simulink model "IEEE13NodeTestFeeder"  (R2024a)
settings: Solver=ode45  StartTime=0.0  StopTime=0.2  MaxStep=0.04  RelTol=1e-3
PreLoadFcn:
  | IEEE13NodeTestFeederInit;
  | Ts=50e-6
undefined symbols (not defined in the file or in its folder): C_601, C_602, C_603, C_604, C_605, C_606, C_607, ft2km, L_601, L_602, L_603, L_604, L_605, L_606, L_607, R_601, R_602, R_603, R_604, R_605, R_606, R_607
libraries: spsLoadFlowBusLib x12, spsPiSectionLineLib x9, spsThreePhaseSeriesRLCLoadLib x7, spsThreePhaseDynamicLoadLib x6, spsGroundLib x6, spsMultimeterLib x6, spsPowerPhasorLib x6, spsSeriesRLCLoadLib x5, spsThreePhaseVIMeasurementLib x4, spsThreePhaseSourceLib x1, spsThreePhaseBreakerLib x1, spsThreePhaseTransformerTwoWindingsLib x1
settings Model: Creator=The MathWorks, Inc.  LastModifiedBy=ethan
settings SolverCC: AlgebraicLoopSolver=TrustRegion
settings DataIOCC: ExternalInput=getinputstruct(op_IEEE_13_node_5)  InitialState=getstatestruct(op_IEEE_13_node_5)  LimitDataPoints=on  SaveFormat=Array  ReturnWorkspaceOutputs=off
settings OptimizationCC: LifeSpan=inf
settings DebuggingCC: AlgebraicLoopMsg=none  FcnCallInpInsideContextMsg=warning  StateNameClashWarn=warning  SFUnexpectedBacktrackingDiag=warning  SFNoUnconditionalDefaultTransitionDiag=warning  SFExecutionAtInitializationDiag=none
settings ModelReferenceCC: EnableRefExpFcnMdlSchedulingChecks=on  PropagateSignalLabelsOutOfModel=off
settings SFSimCC: CustomCodeUndefinedFunction=UseInterfaceOnly
settings RTWCC: GPUComputeCapability=3.5
settings CodeAppCC: StateflowObjectComments=on
settings SimscapeCC: SimscapeNormalizeSystem=off

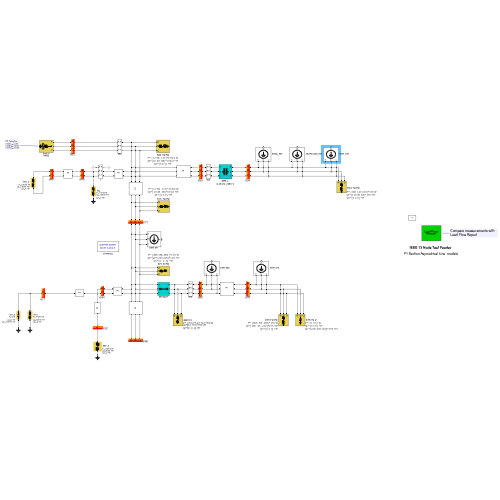
[thumbnail: Simulink's stored preview of the top-level diagram]
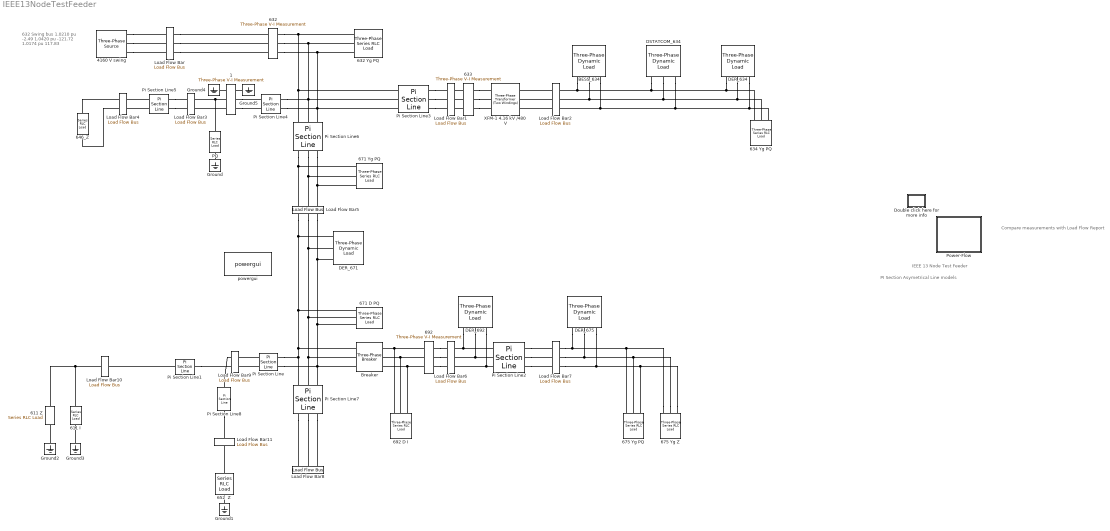
== system IEEE13NodeTestFeeder ==
  note: Compare measurements with
      | Load Flow Report
  note: 632 Swing bus
      | 1.0210 pu -2.49
      | 1.0420 pu -121.72
      | 1.0174 pu 117.83
  note: PI Section Asymetrical Line models
  note: IEEE 13 Node Test Feeder
  " 634 Yg PQ " : spsThreePhaseSeriesRLCLoadLib/Three-Phase Series RLC Load  LConnTagsString=A|B|C  Configuration=Y (grounded)  NominalVoltage=120e3  Vabc=[ 1.04003 1.06954 1.04523]*277.128  Vabcp=[1e3 1e3 1e3]  NominalFrequency=60  UnbalancedPower=on  ActivePower=1e+006  InductivePower=0  CapacitivePower=0  Pabc=[160 120 120]*1e3  QLabc=[110 90 90]*1e3  QCabc=[0 0 0]  Pabcp=[10e3 9e3 11e3]  QLabcp=[100 90 110]  QCabcp=[100 90 110]  Measurements=None  LoadType=constant PQ
      settings: AttributesFormatString=|
      | P= %<Pabc> W
      | Ql=%<QLabc> var
      | Qc=%<QCabc> var
  1 : spsThreePhaseVIMeasurementLib/Three-Phase V-I Measurement  VoltageMeasurement=phase-to-ground  SetLabelV=on  LabelV=Vabc_645  Vpu=off  VpuLL=off  CurrentMeasurement=yes  SetLabelI=on  LabelI=Iabc_645  Ipu=off  Pbase=100e6  Vbase=4160  OutputType=Complex  PhasorSimulation=on  PSBequivalent=0
  4160 V swing : spsThreePhaseSourceLib/Three-Phase Source  InternalConnection=Yg  VoltagePhases=on  Voltage=120e3  PhaseAngle=0  Voltage_phases=[ 1.021 1.042 1.0174]*2401.78  PhaseAngles_phases=[ -2.49008 -121.72 117.83]  Frequency=60  NonIdealSource=on  SpecifyImpedance=off  Resistance=1e-5  Inductance=0  ShortCircuitLevel=100e6  BaseVoltage=120e3  XRratio=10  BusType=swing  Pref=0  Qref=0  Prefabc=[0 0 0]  Qrefabc=[0 0 0]  Qmin="[-inf  -inf -inf]"  Qmax="[inf  inf inf]"
  611 I : spsSeriesRLCLoadLib/Series RLC Load  LConnTagsString=a  RConnTagsString=__new0  NominalVoltage=0.986755*2401.78  NominalFrequency=60  ActivePower=170e3  InductivePower=80e3  CapacitivePower=0  Setx0=off  InitialVoltage=0  SetiL0=off  InitialCurrent=0  Measurements=Branch voltage and current  LoadType=constant I
      settings: AttributesFormatString=|
      | P=%<ActivePower> W
      | Ql=%<InductivePower> var
      | Qc=%<CapacitivePower> var
  611 Z : spsSeriesRLCLoadLib/Series RLC Load  LConnTagsString=a  RConnTagsString=__new0  NominalVoltage=4160/sqrt(3)  NominalFrequency=60  ActivePower=0  InductivePower=0  CapacitivePower=100e3  Setx0=off  InitialVoltage=0  SetiL0=off  InitialCurrent=0  Measurements=None  LoadType=constant Z
      settings: AttributesFormatString=|
      | P=%<ActivePower> W
      | Ql=%<InductivePower> var
      | Qc=%<CapacitivePower> var
  632 : spsThreePhaseVIMeasurementLib/Three-Phase V-I Measurement  VoltageMeasurement=phase-to-ground  SetLabelV=on  LabelV=Vabc_632  Vpu=off  VpuLL=off  CurrentMeasurement=yes  SetLabelI=on  LabelI=Iabc_632  Ipu=off  Pbase=100e6  Vbase=4160  OutputType=Complex  PhasorSimulation=on  PSBequivalent=0
  632 Yg PQ : spsThreePhaseSeriesRLCLoadLib/Three-Phase Series RLC Load  LConnTagsString=A|B|C  Configuration=Y (grounded)  NominalVoltage=120e3  Vabc=[ 1.021 1.042 1.0174]*2401.78  Vabcp=[1e3 1e3 1e3]  NominalFrequency=60  UnbalancedPower=on  ActivePower=1e+006  InductivePower=0  CapacitivePower=0  Pabc="[17 66  117]*1e3/2"  QLabc="[10 38  68]*1e3/2"  QCabc=[0 0 0]  Pabcp=[10e3 9e3 11e3]  QLabcp=[100 90 110]  QCabcp=[100 90 110]  Measurements=None  LoadType=constant PQ
      settings: AttributesFormatString=|
      | P= %<Pabc> W
      | Ql=%<QLabc> var
      | Qc=%<QCabc> var
  633 : spsThreePhaseVIMeasurementLib/Three-Phase V-I Measurement  VoltageMeasurement=phase-to-ground  SetLabelV=on  LabelV=Vabc_633  Vpu=off  VpuLL=off  CurrentMeasurement=yes  SetLabelI=on  LabelI=Iabc_633  Ipu=off  Pbase=100e6  Vbase=4160  OutputType=Complex  PhasorSimulation=on  PSBequivalent=0
  646_Z : spsSeriesRLCLoadLib/Series RLC Load  LConnTagsString=a  RConnTagsString=__new0  NominalVoltage=4160  NominalFrequency=60  ActivePower=230e3  InductivePower=132e3  CapacitivePower=0  Setx0=off  InitialVoltage=0  SetiL0=off  InitialCurrent=0  Measurements=None  LoadType=constant Z
      settings: AttributesFormatString=|
      | P=%<ActivePower> W
      | Ql=%<InductivePower> var
      | Qc=%<CapacitivePower> var
  "652  Z " : spsSeriesRLCLoadLib/Series RLC Load  LConnTagsString=a  RConnTagsString=__new0  NominalVoltage=4160/sqrt(3)  NominalFrequency=60  ActivePower=128e3  InductivePower=86e3  CapacitivePower=0  Setx0=off  InitialVoltage=0  SetiL0=off  InitialCurrent=0  Measurements=None  LoadType=constant Z
      settings: AttributesFormatString=|
      | P=%<ActivePower> W
      | Ql=%<InductivePower> var
      | Qc=%<CapacitivePower> var
  671 D PQ : spsThreePhaseSeriesRLCLoadLib/Three-Phase Series RLC Load  LConnTagsString=A|B|C  Configuration=Delta  NominalVoltage=120e3  Vabc="[1  1  1]*120e3/sqrt(3)"  Vabcp=[ 1.7426 1.77325 1.71534]*2401.78  NominalFrequency=60  UnbalancedPower=on  ActivePower=1e+006  InductivePower=0  CapacitivePower=0  Pabc="[17 66  117]*1e3/2"  QLabc="[10 38  68]*1e3/2"  QCabc=[0 0 0]  Pabcp=[385 385 385 ]*1e3  QLabcp=[220 220 220]*1e3  QCabcp="[0  0  0]"  Measurements=Branch voltages and currents  LoadType=constant PQ
      settings: AttributesFormatString=|
      | P= %<Pabcp> W
      | Ql=%<QLabcp> var
      | Qc=%<QCabcp> var
  671 Yg PQ : spsThreePhaseSeriesRLCLoadLib/Three-Phase Series RLC Load  LConnTagsString=A|B|C  Configuration=Y (grounded)  NominalVoltage=120e3  Vabc=[ 0.990007 1.05293 0.977696]*2401.78  Vabcp=[1e3 1e3 1e3]  NominalFrequency=60  UnbalancedPower=on  ActivePower=1e+006  InductivePower=0  CapacitivePower=0  Pabc="[17 66  117]*1e3/2"  QLabc="[10 38  68]*1e3/2"  QCabc=[0 0 0]  Pabcp=[10e3 9e3 11e3]  QLabcp=[100 90 110]  QCabcp=[100 90 110]  Measurements=None  LoadType=constant PQ
      settings: AttributesFormatString=|
      | P= %<Pabc> W
      | Ql=%<QLabc> var
      | Qc=%<QCabc> var
  675 Yg PQ : spsThreePhaseSeriesRLCLoadLib/Three-Phase Series RLC Load  LConnTagsString=A|B|C  Configuration=Y (grounded)  NominalVoltage=120e3  Vabc=[ 0.983621 1.05532 0.975578]*2401.78  Vabcp=[1e3 1e3 1e3]  NominalFrequency=60  UnbalancedPower=on  ActivePower=1e+006  InductivePower=0  CapacitivePower=0  Pabc="[485  68  290]*1e3"  QLabc="[190  60  212]*1e3"  QCabc=[0 0 0]  Pabcp=[10e3 9e3 11e3]  QLabcp=[100 90 110]  QCabcp=[100 90 110]  Measurements=Branch voltages and currents  LoadType=constant PQ
      settings: AttributesFormatString=|
      | P= %<Pabc> W
      | Ql=%<QLabc> var
      | Qc=%<QCabc> var
  675 Yg Z : spsThreePhaseSeriesRLCLoadLib/Three-Phase Series RLC Load  LConnTagsString=A|B|C  Configuration=Y (grounded)  NominalVoltage=120e3  Vabc="[1  1  1]*4160/sqrt(3)"  Vabcp=[1e3 1e3 1e3]  NominalFrequency=60  UnbalancedPower=on  ActivePower=1e+006  InductivePower=0  CapacitivePower=0  Pabc=[0 0 0]  QLabc=[0 0 0]  QCabc=[200 200 200]*1e3  Pabcp=[10e3 9e3 11e3]  QLabcp=[100 90 110]  QCabcp=[100 90 110]  Measurements=None  LoadType=constant Z
      settings: AttributesFormatString=|
      | P= %<Pabc> W
      | Ql=%<QLabc> var
      | Qc=%<QCabc> var
  692 : spsThreePhaseVIMeasurementLib/Three-Phase V-I Measurement  VoltageMeasurement=phase-to-ground  SetLabelV=on  LabelV=Vabc_692  Vpu=off  VpuLL=off  CurrentMeasurement=yes  SetLabelI=on  LabelI=Iabc_692  Ipu=off  Pbase=100e6  Vbase=4160  OutputType=Complex  PhasorSimulation=on  PSBequivalent=0
  692 D I : spsThreePhaseSeriesRLCLoadLib/Three-Phase Series RLC Load  LConnTagsString=A|B|C  Configuration=Delta  NominalVoltage=120e3  Vabc="[1  1  1]*120e3/sqrt(3)"  Vabcp=[ 1.73731 1.75253 1.72367]*2401.78  NominalFrequency=60  UnbalancedPower=on  ActivePower=1e+006  InductivePower=0  CapacitivePower=0  Pabc="[17 66  117]*1e3/2"  QLabc="[10 38  68]*1e3/2"  QCabc=[0 0 0]  Pabcp=[1e-6 1e-6 170 ]*1e3  QLabcp=[0 0 151]*1e3  QCabcp="[0  0  0]"  Measurements=Branch voltages and currents  LoadType=constant I
      settings: AttributesFormatString=|
      | P= %<Pabcp> W
      | Ql=%<QLabcp> var
      | Qc=%<QCabcp> var
  BESS_634 : spsThreePhaseDynamicLoadLib/Three-Phase Dynamic Load  NominalVoltage=[4160 60]  ActiveReactivePowers=[0 0]  PositiveSequence=[0.121336 5.51821]  ExternalControl=off  NpNq=[0 0]  TimeConstants="[0  0  0  0]"  MinimumVoltage=0.7  Tfilter=1e-4  LoadFlowParameters=[4,0,0,0,0]
      settings: LibrarySourceBlock=|
      | sps_lib/Passives/Three-Phase
      | Dynamic Load
  Breaker : spsThreePhaseBreakerLib/Three-Phase Breaker  InitialState=closed  SwitchA=off  SwitchB=off  SwitchC=off  SwitchTimes=[0.5 ]  External=off  BreakerResistance=0.0001  SnubberResistance=inf  SnubberCapacitance=0  Measurements=None
  DER_634 : spsThreePhaseDynamicLoadLib/Three-Phase Dynamic Load  NominalVoltage=[4160 60]  ActiveReactivePowers=[0 0]  PositiveSequence=[0.121336 5.51821]  ExternalControl=off  NpNq=[0 0]  TimeConstants="[0  0  0  0]"  MinimumVoltage=0.7  Tfilter=1e-4  LoadFlowParameters=[4,0,0,0,0]
      settings: LibrarySourceBlock=|
      | sps_lib/Passives/Three-Phase
      | Dynamic Load
  DER_671 : spsThreePhaseDynamicLoadLib/Three-Phase Dynamic Load  NominalVoltage=[4160 60]  ActiveReactivePowers=[0 0]  PositiveSequence=[1.00665 -3.83837]  ExternalControl=off  NpNq=[0 0]  TimeConstants="[0  0  0  0]"  MinimumVoltage=0.7  Tfilter=1e-4  LoadFlowParameters=[4,0,0,0,0]
      settings: LibrarySourceBlock=|
      | sps_lib/Passives/Three-Phase
      | Dynamic Load
  DER_675 : spsThreePhaseDynamicLoadLib/Three-Phase Dynamic Load  NominalVoltage=[4160 60]  ActiveReactivePowers=[0 0]  PositiveSequence=[1.0046 -3.96901]  ExternalControl=off  NpNq=[0 0]  TimeConstants="[0  0  0  0]"  MinimumVoltage=0.7  Tfilter=1e-4  LoadFlowParameters=[4,0,0,0,0]
      settings: LibrarySourceBlock=|
      | sps_lib/Passives/Three-Phase
      | Dynamic Load
  DER_692 : spsThreePhaseDynamicLoadLib/Three-Phase Dynamic Load  NominalVoltage=[4160 60]  ActiveReactivePowers=[0 0]  PositiveSequence=[1.00665 -3.83836]  ExternalControl=off  NpNq=[0 0]  TimeConstants="[0  0  0  0]"  MinimumVoltage=0.7  Tfilter=1e-4  LoadFlowParameters=[4,0,0,0,0]
      settings: LibrarySourceBlock=|
      | sps_lib/Passives/Three-Phase
      | Dynamic Load
  DSTATCOM_634 : spsThreePhaseDynamicLoadLib/Three-Phase Dynamic Load  NominalVoltage=[4160 60]  ActiveReactivePowers=[0 0]  PositiveSequence=[0.121336 5.51821]  ExternalControl=off  NpNq=[0 0]  TimeConstants="[0  0  0  0]"  MinimumVoltage=0.7  Tfilter=1e-4  LoadFlowParameters=[4,0,0,0,0]
      settings: LibrarySourceBlock=|
      | sps_lib/Passives/Three-Phase
      | Dynamic Load
  Double click here for more info : Subsystem
      settings: OpenFcn="showExample(\"simscapeelectricalsps/IEEE13NodeTestFeederExample\")"
      mask Display: disp('?')
  Ground{,1..5} (6 alike) : spsGroundLib/Ground  LConnTagsString=a
  Load Flow Bar : spsLoadFlowBusLib/Load Flow Bus  LConnTagsString=a|b|c  RConnTagsString=a|b|c  Phases=ABC  Connectors=on both sides  ID=632  Vbase=4160/sqrt(3)  Vref="[ 1.0210  1.0420  1.0174]"  Vangle="[ -2.49  -121.72  117.83]"  VLF=1.021  VLFb=1.042  VLFc=1.017  angleLF=-2.49  angleLFb=-121.7  angleLFc=117.8
      settings: AttributesFormatString=%<ID>
  Load Flow Bar1 : spsLoadFlowBusLib/Load Flow Bus  LConnTagsString=a|b|c  RConnTagsString=a|b|c  Phases=ABC  Connectors=on both sides  ID=633  Vbase=4160/sqrt(3)  Vref=[1.0 1.0 1.0]  Vangle=[0 -120 120]  VLF=1.023  VLFb=1.046  VLFc=1.023  angleLF=-1.782  angleLFb=-120.9  angleLFc=118.7
      settings: AttributesFormatString=%<ID>
  Load Flow Bar10 : spsLoadFlowBusLib/Load Flow Bus  LConnTagsString=a  RConnTagsString=a  Phases=C  Connectors=on both sides  ID=611  Vbase=4160/sqrt(3)  Vref=1.0  Vangle=0  VLF=NaN  VLFb=NaN  VLFc=0.9737  angleLF=NaN  angleLFb=NaN  angleLFc=115.8
      settings: AttributesFormatString=%<ID>
  Load Flow Bar11 : spsLoadFlowBusLib/Load Flow Bus  LConnTagsString=a  RConnTagsString=a  Phases=A  Connectors=on both sides  ID=652  Vbase=4160/sqrt(3)  Vref=1.0  Vangle=0  VLF=0.9825  VLFb=NaN  VLFc=NaN  angleLF=-5.246  angleLFb=NaN  angleLFc=NaN
      settings: AttributesFormatString=%<ID>
  Load Flow Bar2 : spsLoadFlowBusLib/Load Flow Bus  LConnTagsString=a|b|c  RConnTagsString=a|b|c  Phases=ABC  Connectors=on both sides  ID=634  Vbase=480/sqrt(3)  Vref=[1.0 1.0 1.0]  Vangle=[0 -120 120]  VLF=1.04  VLFb=1.07  VLFc=1.045  angleLF=5.014  angleLFb=-114.1  angleLFc=125.6
      settings: AttributesFormatString=%<ID>
  Load Flow Bar3 : spsLoadFlowBusLib/Load Flow Bus  LConnTagsString=a|b  RConnTagsString=a|b  Phases=BC  Connectors=on both sides  ID=645  Vbase=4160/sqrt(3)  Vref=[1.0 1.0 ]  Vangle=[0 0]  VLF=NaN  VLFb=1.033  VLFc=1.015  angleLF=NaN  angleLFb=-121.9  angleLFc=117.9
      settings: AttributesFormatString=%<ID>
  Load Flow Bar4 : spsLoadFlowBusLib/Load Flow Bus  LConnTagsString=a|b  RConnTagsString=a|b  Phases=BC  Connectors=on both sides  ID=646  Vbase=4160/sqrt(3)  Vref=[1.0 1.0 ]  Vangle=[0 0]  VLF=NaN  VLFb=1.031  VLFc=1.013  angleLF=NaN  angleLFb=-122  angleLFc=117.9
      settings: AttributesFormatString=%<ID>
  Load Flow Bar5 : spsLoadFlowBusLib/Load Flow Bus  LConnTagsString=a|b|c  RConnTagsString=a|b|c  Phases=ABC  Connectors=on both sides  ID=671  Vbase=4160/sqrt(3)  Vref=[1.0 1.0 1.0]  Vangle=[0 -120 120]  VLF=0.99  VLFb=1.053  VLFc=0.9777  angleLF=-5.298  angleLFb=-122.3  angleLFc=116
      settings: AttributesFormatString=%<ID>
  Load Flow Bar6 : spsLoadFlowBusLib/Load Flow Bus  LConnTagsString=a|b|c  RConnTagsString=a|b|c  Phases=ABC  Connectors=on both sides  ID=692  Vbase=4160/sqrt(3)  Vref=[1.0 1.0 1.0]  Vangle=[0 -120 120]  VLF=0.99  VLFb=1.053  VLFc=0.9777  angleLF=-5.298  angleLFb=-122.3  angleLFc=116
      settings: AttributesFormatString=%<ID>
  Load Flow Bar7 : spsLoadFlowBusLib/Load Flow Bus  LConnTagsString=a|b|c  RConnTagsString=a|b|c  Phases=ABC  Connectors=on both sides  ID=675  Vbase=4160/sqrt(3)  Vref=[1.0 1.0 1.0]  Vangle=[0 -120 120]  VLF=0.9836  VLFb=1.055  VLFc=0.9756  angleLF=-5.544  angleLFb=-122.5  angleLFc=116
      settings: AttributesFormatString=%<ID>
  Load Flow Bar8 : spsLoadFlowBusLib/Load Flow Bus  LConnTagsString=a|b|c  Phases=ABC  Connectors=on one side  ID=680  Vbase=4160/sqrt(3)  Vref=[1.0 1.0 1.0]  Vangle=[0 -120 120]  VLF=0.99  VLFb=1.053  VLFc=0.9777  angleLF=-5.298  angleLFb=-122.3  angleLFc=116
      settings: AttributesFormatString=%<ID>
  Load Flow Bar9 : spsLoadFlowBusLib/Load Flow Bus  LConnTagsString=a|b  RConnTagsString=a|b  Phases=AC  Connectors=on both sides  ID=684  Vbase=4160/sqrt(3)  Vref=[1.0 1.0 ]  Vangle=[0 -120 ]  VLF=0.9881  VLFb=NaN  VLFc=0.9757  angleLF=-5.321  angleLFb=NaN  angleLFc=115.9
      settings: AttributesFormatString=%<ID>
  PQ : spsSeriesRLCLoadLib/Series RLC Load  LConnTagsString=a  RConnTagsString=__new0  NominalVoltage=1.03283*2401.78  NominalFrequency=60  ActivePower=170e3  InductivePower=125e3  CapacitivePower=0  Setx0=off  InitialVoltage=0  SetiL0=off  InitialCurrent=0  Measurements=None  LoadType=constant PQ
      settings: AttributesFormatString=|
      | P=%<ActivePower> W
      | Ql=%<InductivePower> var
      | Qc=%<CapacitivePower> var
  Pi Section Line : spsPiSectionLineLib/Pi Section Line  LConnTagsString=1|i2  RConnTagsString=1|o2  Phases=2  PiSections=1  Length=300*ft2km  Frequency=60  Resistance=R_604([1 3],[1 3])  Inductance=L_604([1 3],[1 3])  Capacitance=C_604([1 3],[1 3])  SpecifyConductance=off  Conductance=0  Measurements=None  Measurements2=None
      settings: LibrarySourceBlock=sps_lib/Power Grid Elements/Pi Section Line
  Pi Section Line1 : spsPiSectionLineLib/Pi Section Line  LConnTagsString=1  RConnTagsString=1  Phases=1  PiSections=1  Length=300*ft2km  Frequency=60  Resistance=R_605(3,3)  Inductance=L_605(3,3)  Capacitance=C_605(3,3)  SpecifyConductance=off  Conductance=0  Measurements=None  Measurements2=None
      settings: LibrarySourceBlock=sps_lib/Power Grid Elements/Pi Section Line
  Pi Section Line2 : spsPiSectionLineLib/Pi Section Line  LConnTagsString=1|i2|i3  RConnTagsString=1|o2|o3  Phases=3  PiSections=1  Length=500*ft2km  Frequency=60  Resistance=R_606  Inductance=L_606  Capacitance=C_606  SpecifyConductance=off  Conductance=0  Measurements=None  Measurements2=None
      settings: LibrarySourceBlock=sps_lib/Power Grid Elements/Pi Section Line
  Pi Section Line3 : spsPiSectionLineLib/Pi Section Line  LConnTagsString=1|i2|i3  RConnTagsString=1|o2|o3  Phases=3  PiSections=1  Length=500*ft2km  Frequency=60  Resistance=R_602  Inductance=L_602  Capacitance=C_602  SpecifyConductance=off  Conductance=0  Measurements=None  Measurements2=None
      settings: LibrarySourceBlock=sps_lib/Power Grid Elements/Pi Section Line
  Pi Section Line4 : spsPiSectionLineLib/Pi Section Line  LConnTagsString=1|i2  RConnTagsString=1|o2  Phases=2  PiSections=1  Length=500*ft2km  Frequency=60  Resistance=R_603(2:3,2:3)  Inductance=L_603(2:3,2:3)  Capacitance=C_603(2:3,2:3)  SpecifyConductance=off  Conductance=0  Measurements=None  Measurements2=None
      settings: LibrarySourceBlock=sps_lib/Power Grid Elements/Pi Section Line
  Pi Section Line5 : spsPiSectionLineLib/Pi Section Line  LConnTagsString=1|i2  RConnTagsString=1|o2  Phases=2  PiSections=1  Length=300*ft2km  Frequency=60  Resistance=R_603(2:3,2:3)  Inductance=L_603(2:3,2:3)  Capacitance=C_603(2:3,2:3)  SpecifyConductance=off  Conductance=0  Measurements=None  Measurements2=None
      settings: LibrarySourceBlock=sps_lib/Power Grid Elements/Pi Section Line
  Pi Section Line6 : spsPiSectionLineLib/Pi Section Line  LConnTagsString=1|i2|i3  RConnTagsString=1|o2|o3  Phases=3  PiSections=1  Length=2000*ft2km  Frequency=60  Resistance=R_601  Inductance=L_601  Capacitance=C_601  SpecifyConductance=off  Conductance=0  Measurements=None  Measurements2=None
      settings: LibrarySourceBlock=sps_lib/Power Grid Elements/Pi Section Line
  Pi Section Line7 : spsPiSectionLineLib/Pi Section Line  LConnTagsString=1|i2|i3  RConnTagsString=1|o2|o3  Phases=3  PiSections=1  Length=1000*ft2km  Frequency=60  Resistance=R_601  Inductance=L_601  Capacitance=C_601  SpecifyConductance=off  Conductance=0  Measurements=None  Measurements2=None
      settings: LibrarySourceBlock=sps_lib/Power Grid Elements/Pi Section Line
  Pi Section Line8 : spsPiSectionLineLib/Pi Section Line  LConnTagsString=1  RConnTagsString=1  Phases=1  PiSections=1  Length=800*ft2km  Frequency=60  Resistance=R_607(1,1)  Inductance=L_607(1,1)  Capacitance=C_607(1,1)  SpecifyConductance=off  Conductance=0  Measurements=None  Measurements2=None
      settings: LibrarySourceBlock=sps_lib/Power Grid Elements/Pi Section Line
  Power-Flow : Subsystem
      mask Display: disp('Load Flow\nResults')
  XFM-1 4.16 kV /480 V : spsThreePhaseTransformerTwoWindingsLib/Three-Phase Transformer (Two Windings)  Winding1Connection=Yg  Winding2Connection=Yg  CoreType=Three single-phase transformers  SetSaturation=off  Hysteresis=off  DataFile='hysteresis'  SetInitialFlux=off  Measurements=None  UNITS=pu  NominalPower=[ 500e3 , 60 ]  Winding1=[4160 0.011 0.02]  Winding2=[480 0 0]  Rm=500  Lm=500  L0=0.5  Saturation=[0 0;0.0024 1.2;1 1.52]  InitialFluxes=[0.8 -0.8 0.7]  BreakLoop=off  DiscreteSolver=Trapezoidal iterative  DataType=off  TransfoNumber=1
  powergui : spspowerguiLib/powergui  Priority=1  SimulationMode=Discrete phasor  SampleTime=4e-3  frequency=60  Iterations=50  frequencyindice=60  Pbase=100e3  ErrMax=0.0001  UnitsV=kV  UnitsW=kW  buscounter=0  FunctionMessages=off  echomessages=off  EnableUseOfTLC=off  CurrentSourceSwitches=off  DisableSnubberDevices=off  DisableRonSwitches=off  DisableVfSwitches=off  DisplayEquations=off  AutomaticDiscreteSolvers=off  SolverType=Tustin/Backward Euler (TBE)  Interpol=off  ExternalGateDelay=off  methode=off  Ts=0  x0status=blocks  SPID=off  SwTol=0  HookPort=off  NonlinearTolerance=1e-4  nMaxIteration=100  ContinueOnMaxIteration=off  RestoreLinks=warning  ResistiveCurrentMeasurement=off  Frange=[0:2:500]  Ylog=off  Xlog=on  ShowGrid=off  save=off  variable=ZData  structure=0  ZoomFFT=on  StartTime=0.0  cycles=1  DisplayStyle=1  fundamental=60  FreqAxis=off  MaxFrequency=1000  frequencyindicesteady=1  RmsSteady=1  display=off
  connections:
  632/RConn2 -- 632 Yg PQ/LConn2 -- Pi Section Line4/RConn1 -- Pi Section Line6/LConn2 -- Pi Section Line3/LConn2
  675 Yg Z/LConn1 -- DER_675/LConn1 -- Load Flow Bar7/LConn1 -- 675 Yg PQ/LConn1
  671 D PQ/LConn2 -- DER_671/LConn2 -- Load Flow Bar5/RConn2 -- Breaker/LConn2 -- Pi Section Line7/LConn2
  Breaker/RConn3 -- 692 D I/LConn3 -- 692/LConn3
  Pi Section Line/RConn1 -- Pi Section Line7/LConn1 -- DER_671/LConn1 -- Load Flow Bar5/RConn1 -- 671 D PQ/LConn1 -- Breaker/LConn1
  Load Flow Bar3/RConn1 -- 1/LConn2 -- PQ/LConn1
  675 Yg Z/LConn3 -- DER_675/LConn3 -- Load Flow Bar7/LConn3 -- 675 Yg PQ/LConn3
  671 Yg PQ/LConn2 -- Load Flow Bar5/LConn2 -- Pi Section Line6/RConn2
  611 I/LConn1 -- Load Flow Bar10/LConn1 -- 611 Z/LConn1
  671 Yg PQ/LConn3 -- Load Flow Bar5/LConn3 -- Pi Section Line6/RConn3
  Pi Section Line6/LConn1 -- 632 Yg PQ/LConn1 -- 632/RConn1 -- Pi Section Line3/LConn1
  671 D PQ/LConn3 -- DER_671/LConn3 -- Load Flow Bar5/RConn3 -- Pi Section Line7/LConn3 -- Breaker/LConn3 -- Pi Section Line/RConn2
  632/RConn3 -- 632 Yg PQ/LConn3 -- Pi Section Line4/RConn2 -- Pi Section Line6/LConn3 -- Pi Section Line3/LConn3
  Breaker/RConn1 -- 692 D I/LConn1 -- 692/LConn1
  671 Yg PQ/LConn1 -- Load Flow Bar5/LConn1 -- Pi Section Line6/RConn1
  Breaker/RConn2 -- 692 D I/LConn2 -- 692/LConn2
  675 Yg Z/LConn2 -- Load Flow Bar7/LConn2 -- DER_675/LConn2 -- 675 Yg PQ/LConn2
  692/RConn1 -- Load Flow Bar6/RConn1
  1/LConn3 -- Load Flow Bar3/RConn2
  Ground2/LConn1 -- 611 Z/RConn1
  Pi Section Line1/LConn1 -- Load Flow Bar10/RConn1
  692/RConn3 -- Load Flow Bar6/RConn3
  Pi Section Line5/RConn1 -- Load Flow Bar3/LConn1
  Load Flow Bar2/LConn2 -- XFM-1 4.16 kV /480 V/RConn2
  " 634 Yg PQ "/LConn2 -- BESS_634/LConn2 -- Load Flow Bar2/RConn2 -- DSTATCOM_634/LConn2 -- DER_634/LConn2
  4160 V swing/RConn2 -- Load Flow Bar/LConn2
  Pi Section Line2/RConn3 -- Load Flow Bar7/RConn3
  Pi Section Line7/RConn3 -- Load Flow Bar8/LConn3
  Pi Section Line5/RConn2 -- Load Flow Bar3/LConn2
  633/LConn1 -- Load Flow Bar1/RConn1
  Pi Section Line2/RConn1 -- Load Flow Bar7/RConn1
  Ground/LConn1 -- PQ/RConn1
  Pi Section Line/LConn1 -- Load Flow Bar9/RConn1
  Pi Section Line7/RConn1 -- Load Flow Bar8/LConn1
  Load Flow Bar4/LConn2 -- 646_Z/RConn1
  1/RConn3 -- Pi Section Line4/LConn2
  Pi Section Line5/LConn1 -- Load Flow Bar4/RConn1
  Pi Section Line7/RConn2 -- Load Flow Bar8/LConn2
  Pi Section Line8/LConn1 -- Load Flow Bar9/LConn1
  692/RConn2 -- Load Flow Bar6/RConn2
  Ground1/LConn1 -- "652  Z "/RConn1
  Pi Section Line2/LConn1 -- DER_692/LConn1 -- Load Flow Bar6/LConn1
  4160 V swing/RConn1 -- Load Flow Bar/LConn1
  Pi Section Line/LConn2 -- Load Flow Bar9/RConn2
  633/RConn3 -- XFM-1 4.16 kV /480 V/LConn3
  Pi Section Line8/RConn1 -- Load Flow Bar11/LConn1
  4160 V swing/RConn3 -- Load Flow Bar/LConn3
  "652  Z "/LConn1 -- Load Flow Bar11/RConn1
  633/RConn2 -- XFM-1 4.16 kV /480 V/LConn2
  1/RConn1 -- Ground5/LConn1
  633/RConn1 -- XFM-1 4.16 kV /480 V/LConn1
  Pi Section Line2/LConn2 -- DER_692/LConn2 -- Load Flow Bar6/LConn2
  Load Flow Bar/RConn2 -- 632/LConn2
  Ground3/LConn1 -- 611 I/RConn1
  Pi Section Line3/RConn1 -- Load Flow Bar1/LConn1
  Load Flow Bar/RConn1 -- 632/LConn1
  Pi Section Line5/LConn2 -- Load Flow Bar4/RConn2
  Pi Section Line2/RConn2 -- Load Flow Bar7/RConn2
  Pi Section Line3/RConn2 -- Load Flow Bar1/LConn2
  633/LConn3 -- Load Flow Bar1/RConn3
  Load Flow Bar/RConn3 -- 632/LConn3
  Pi Section Line3/RConn3 -- Load Flow Bar1/LConn3
  633/LConn2 -- Load Flow Bar1/RConn2
  Ground4/LConn1 -- 1/LConn1
  Pi Section Line1/RConn1 -- Load Flow Bar9/LConn2
  Load Flow Bar2/LConn1 -- XFM-1 4.16 kV /480 V/RConn1
  " 634 Yg PQ "/LConn1 -- BESS_634/LConn1 -- Load Flow Bar2/RConn1 -- DSTATCOM_634/LConn1 -- DER_634/LConn1
  Pi Section Line2/LConn3 -- DER_692/LConn3 -- Load Flow Bar6/LConn3
  Load Flow Bar2/LConn3 -- XFM-1 4.16 kV /480 V/RConn3
  1/RConn2 -- Pi Section Line4/LConn1
  " 634 Yg PQ "/LConn3 -- BESS_634/LConn3 -- Load Flow Bar2/RConn3 -- DSTATCOM_634/LConn3 -- DER_634/LConn3
  646_Z/LConn1 -- Load Flow Bar4/LConn1

== system IEEE13NodeTestFeeder/Double click here for more info ==

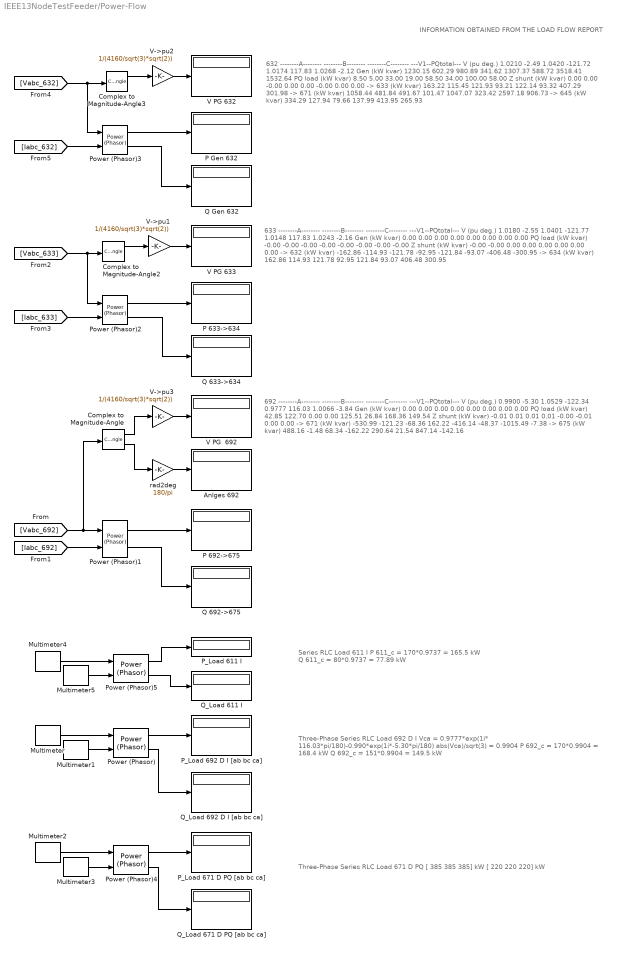
== system IEEE13NodeTestFeeder/Power-Flow ==
  note: 692 --------A-------- --------B-------- --------C-------- ---V1--PQtotal---
      | V (pu deg.) 0.9900 -5.30 1.0529 -122.34 0.9777 116.03 1.0066 -3.84
      | Gen (kW kvar) 0.00 0.00 0.00 0.00 0.00 0.00 0.00 0.00
      | PQ load (kW kvar) 42.85 122.70 0.00 0.00 125.51 26.84 168.36 149.54
      | Z shunt (kW kvar) -0.01 0.01 0.01 0.01 -0.00 -0.01 0.00 0.00
      |
      | -> 671 (kW kvar) -530.99 -121.23 -68.36 162.22 -416.14 -48.37 -1015.49 -7.38
      | -> 675 (kW kvar) 488.16 -1.48 68.34 -162.22 290.64 21.54 847.14 -142.16
  note: 633 --------A-------- --------B-------- --------C-------- ---V1--PQtotal---
      | V (pu deg.) 1.0180 -2.55 1.0401 -121.77 1.0148 117.83 1.0243 -2.16
      | Gen (kW kvar) 0.00 0.00 0.00 0.00 0.00 0.00 0.00 0.00
      | PQ load (kW kvar) -0.00 -0.00 -0.00 -0.00 -0.00 -0.00 -0.00 -0.00
      | Z shunt (kW kvar) -0.00 -0.00 0.00 0.00 0.00 0.00 0.00 0.00
      |
      | -> 632 (kW kvar) -162.86 -114.93 -121.78 -92.95 -121.84 -93.07 -406.48 -300.95
      | -> 634 (kW kvar) 162.86 114.93 121.78 92.95 121.84 93.07 406.48 300.95
  note: 632 --------A-------- --------B-------- --------C-------- ---V1--PQtotal---
      | V (pu deg.) 1.0210 -2.49 1.0420 -121.72 1.0174 117.83 1.0268 -2.12
      | Gen (kW kvar) 1230.15 602.29 980.89 341.62 1307.37 588.72 3518.41 1532.64
      | PQ load (kW kvar) 8.50 5.00 33.00 19.00 58.50 34.00 100.00 58.00
      | Z shunt (kW kvar) 0.00 0.00 -0.00 0.00 0.00 -0.00 0.00 0.00
      |
      | -> 633 (kW kvar) 163.22 115.45 121.93 93.21 122.14 93.32 407.29 301.98
      | -> 671 (kW kvar) 1058.44 481.84 491.67 101.47 1047.07 323.42 2597.18 906.73
      | -> 645 (kW kvar) 334.29 127.94 79.66 137.99 413.95 265.93
  note: Three-Phase Series RLC Load 671 D PQ
      | [ 385 385 385] kW
      | [ 220 220 220] kW
  note: Three-Phase Series RLC Load 692 D I
      | Vca = 0.9777*exp(1i* 116.03*pi/180)-0.990*exp(1i*-5.30*pi/180)
      | abs(Vca)/sqrt(3) = 0.9904
      | P 692_c = 170*0.9904 = 168.4 kW
      | Q 692_c = 151*0.9904 = 149.5 kW
  note: Series RLC Load 611 I
      | P 611_c = 170*0.9737 = 165.5 kW
      | Q 611_c = 80*0.9737 = 77.89 kW
  note: INFORMATION OBTAINED FROM THE LOAD FLOW REPORT
  Anlges 692 : Display
  Complex to Magnitude-Angle : ComplexToMagnitudeAngle
  Complex to Magnitude-Angle2 : ComplexToMagnitudeAngle
  Complex to Magnitude-Angle3 : ComplexToMagnitudeAngle
  Multimeter : spsMultimeterLib/Multimeter  L=20  sel=[8 9 10]  yselected={}  Gain=[1 1 1]  OutputType=Complex  PlotAtSimulationStop=off  PhasorSimulation=on
  Multimeter1 : spsMultimeterLib/Multimeter  L=20  sel=[18 19 20]  yselected={}  Gain=[1 1 1]  OutputType=Complex  PlotAtSimulationStop=off  PhasorSimulation=on
  Multimeter2 : spsMultimeterLib/Multimeter  L=20  sel=[2 3 4]  yselected={}  Gain=[1 1 1]  OutputType=Complex  PlotAtSimulationStop=off  PhasorSimulation=on
  Multimeter3 : spsMultimeterLib/Multimeter  L=20  sel=[12 13 14]  yselected={}  Gain=[1 1 1]  OutputType=Complex  PlotAtSimulationStop=off  PhasorSimulation=on
  Multimeter4 : spsMultimeterLib/Multimeter  L=20  sel=1  yselected={}  Gain=1  OutputType=Complex  PlotAtSimulationStop=off  PhasorSimulation=on
  Multimeter5 : spsMultimeterLib/Multimeter  L=20  sel=11  yselected={}  Gain=1  OutputType=Complex  PlotAtSimulationStop=off  PhasorSimulation=on
  P 633->634 : Display
  P 692->675 : Display
  P Gen 632 : Display
  P_Load 611 I : Display
  P_Load 671 D PQ [ab bc ca] : Display
  P_Load 692 D I [ab bc ca] : Display
  Power (Phasor){,1..5} (6 alike) : spsPowerPhasorLib/Power (Phasor)
      settings: LibrarySourceBlock=|
      | sps_lib/Sensors and Measurements/Power
      | (Phasor)
  Q 633->634 : Display
  Q 692->675 : Display
  Q Gen 632 : Display
  Q_Load 611 I : Display
  Q_Load 671 D PQ [ab bc ca] : Display
  Q_Load 692 D I [ab bc ca] : Display
  V PG  692 : Display
  V PG 632 : Display
  V PG 633 : Display
  V->pu1 : Gain  Gain=1/(4160/sqrt(3)*sqrt(2))
  V->pu2 : Gain  Gain=1/(4160/sqrt(3)*sqrt(2))
  V->pu3 : Gain  Gain=1/(4160/sqrt(3)*sqrt(2))
  rad2deg : Gain  Gain=180/pi
  wires:
  V->pu3/1 -> V PG  692/1
  Power (Phasor)5/2 -> Q_Load 611 I/1
  Power (Phasor)5/1 -> P_Load 611 I/1
  Multimeter5/1 -> Power (Phasor)5/2
  Multimeter4/1 -> Power (Phasor)5/1
  rad2deg/1 -> Anlges 692/1
  Complex to Magnitude-Angle/2 -> rad2deg/1
  [Vabc_692] -> Complex to Magnitude-Angle/1, Power (Phasor)1/1
  Complex to Magnitude-Angle/1 -> V->pu3/1
  Power (Phasor)4/2 -> Q_Load 671 D PQ [ab bc ca]/1
  Power (Phasor)4/1 -> P_Load 671 D PQ [ab bc ca]/1
  Multimeter3/1 -> Power (Phasor)4/2
  Multimeter2/1 -> Power (Phasor)4/1
  Power (Phasor)/2 -> Q_Load 692 D I [ab bc ca]/1
  Power (Phasor)/1 -> P_Load 692 D I [ab bc ca]/1
  Multimeter1/1 -> Power (Phasor)/2
  Multimeter/1 -> Power (Phasor)/1
  V->pu2/1 -> V PG 632/1
  [Vabc_632] -> Complex to Magnitude-Angle3/1, Power (Phasor)3/1
  Complex to Magnitude-Angle3/1 -> V->pu2/1
  Power (Phasor)3/2 -> Q Gen 632/1
  Power (Phasor)3/1 -> P Gen 632/1
  [Iabc_632] -> Power (Phasor)3/2
  V->pu1/1 -> V PG 633/1
  [Vabc_633] -> Complex to Magnitude-Angle2/1, Power (Phasor)2/1
  Complex to Magnitude-Angle2/1 -> V->pu1/1
  Power (Phasor)2/2 -> Q 633->634/1
  Power (Phasor)2/1 -> P 633->634/1
  [Iabc_633] -> Power (Phasor)2/2
  Power (Phasor)1/2 -> Q 692->675/1
  Power (Phasor)1/1 -> P 692->675/1
  [Iabc_692] -> Power (Phasor)1/2
